simulink model "ATABEY_Model_sim"  (R2025b)
settings: Solver=VariableStepAuto  StartTime=0.0  StopTime=simTime  RelTol=1e-3
undefined symbols (not defined in the file or in its folder): x0
libraries: aerolibfltsims x2, instrumentseriallib x2, slpidlib x1
settings Model: Creator=erayacikgz  LastModifiedBy=Qeyosa

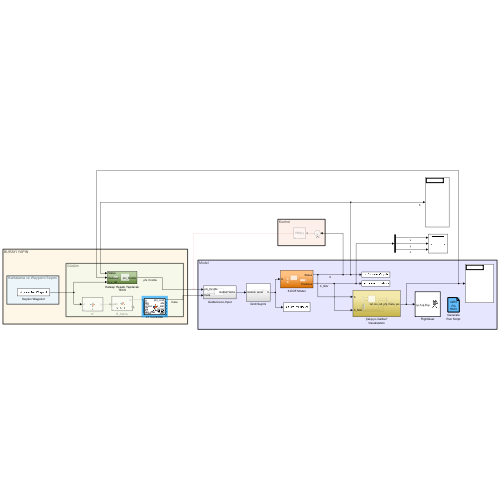
[thumbnail: Simulink's stored preview of the top-level diagram]
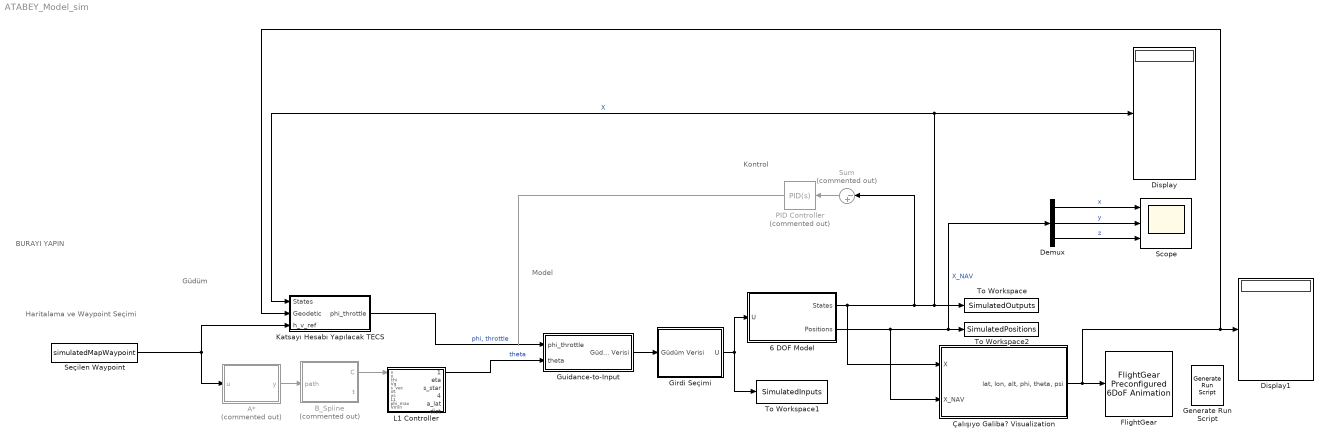
== system ATABEY_Model_sim ==
  note: BURAYI YAPIN
  note: Kontrol
  note: Haritalama ve Waypoint Seçimi
  note: Güdüm
  note: Model
  6 DOF Model : Subsystem
  A* : MATLAB Function  Commented=on  TreatAsAtomicUnit=on
  B_Spline : MATLAB Function  Commented=on  TreatAsAtomicUnit=on
  Demux : Demux  Outputs=3
  Display : Display
  Display1 : Display
  "FlightGear " : aerolibfltsims/FlightGear Preconfigured 6DoF Animation  xFlightGearVersion=v2019.1  DestinationIpAddress=127.0.0.1  DestinationPort=5502  SampleTime=1/30  packetVersion=24
  Generate Run Script : aerolibfltsims/Generate Run Script  Architecture=Linux  dataFlow=Send  GeometryModelName=c172p  AirportId=KSFO  RunwayId=10L  InitialAltitude=7224  InitialHeading=113  OffsetDistance=4.72  OffsetAzimuth=0  InstallScenery=off  DisableShaders=on  OriginAddress=127.0.0.1  DestinationPort=5502  OriginPort=5505  LocalAddress=127.0.0.1  OutputFileName=runfg.sh  FlightGearBaseDirectory=/usr/share/games/flightgear/
  Girdi Seçimi : Subsystem
  Guidance-to-Input : Subsystem
  Katsayı Hesabı Yapılacak TECS : Subsystem
  L1 Controller : MATLAB Function  TreatAsAtomicUnit=on
  PID Controller : slpidlib/PID Controller  Commented=on  Controller=PID  Form=Parallel  TimeDomain=Continuous-time  UseExternalTs=off  SampleTime=-1  IntegratorMethod=Forward Euler  FilterMethod=Forward Euler  ControllerParametersSource=internal  P=1  I=1  UseKiTs=off  D=0  UseExternalDerivativeSource=off  N=100  UseFilter=on  TunerSelectOption=Transfer Function Based (PID Tuner App)  InitialConditionSource=internal  InitialConditionForIntegrator=0  InitialConditionForFilter=0  DifferentiatorICPrevScaledInput=0  ExternalReset=none  TrackingMode=off  Kt=1  LimitOutput=off  SatLimitsSource=internal  UpperSaturationLimit=inf  LowerSaturationLimit=-inf  LinearizeAsGain=on  AntiWindupMode=none  Kb=1  LimitIntegrator=off  UpperIntegratorSaturationLimit=inf  LowerIntegratorSaturationLimit=-inf  POutMin=[]  POutMax=[]  IOutMin=[]  IOutMax=[]  DOutMin=[]  DOutMax=[]  NOutMin=[]  NOutMax=[]  SumOutMin=[]  SumOutMax=[]  SaturationOutMin=[]  SaturationOutMax=[]  PParamMin=[]  PParamMax=[]  IParamMin=[]  IParamMax=[]  DParamMin=[]  DParamMax=[]  NParamMin=[]  NParamMax=[]  KbParamMin=[]  KbParamMax=[]  KtParamMin=[]  KtParamMax=[]  KbOutMin=[]  KbOutMax=[]  KtOutMin=[]  KtOutMax=[]  IntegratorOutMin=[]  IntegratorOutMax=[]  FilterOutMin=[]  FilterOutMax=[]  SumI1OutMin=[]  SumI1OutMax=[]  SumI2OutMin=[]  SumI2OutMax=[]  SumI3OutMin=[]  SumI3OutMax=[]  SumI4OutMin=[]  SumI4OutMax=[]  SumDOutMin=[]  SumDOutMax=[]  DifferentiatorOutMin=[]  DifferentiatorOutMax=[]  FilterDiffOutCoefMin=[]  FilterDiffOutCoefMax=[]  ReciprocalOutMin=[]  ReciprocalOutMax=[]  SumDenOutMin=[]  SumDenOutMax=[]  SumNumOutMin=[]  SumNumOutMax=[]  DivideOutMin=[]  DivideOutMax=[]  UdiffTsProdOutMin=[]  UdiffTsProdOutMax=[]  NTsProdOutMin=[]  NTsProdOutMax=[]  UintegralTsProdOutMin=[]  UintegralTsProdOutMax=[]  UngainTsProdOutMin=[]  UngainTsProdOutMax=[]  ClampingZeroOutDataTypeStr=Inherit: Inherit via back propagation  ClampingZeroOutMin=[]  ClampingZeroOutMax=[]  FilterDenConstantOutDataTypeStr=Inherit: Inherit via back propagation  FilterDenConstantOutMin=[]  FilterDenConstantOutMax=[]  PCopyOutDataTypeStr=Inherit: Inherit via back propagation  PCopyOutMin=[]  PCopyOutMax=[]  NCopyOutDataTypeStr=Inherit: Inherit via back propagation  NCopyOutMin=[]  NCopyOutMax=[]  IntegratorContinuousStateAttributes=''  IntegratorStateMustResolveToSignalObject=off  IntegratorRTWStateStorageClass=Auto  FilterContinuousStateAttributes=''  FilterStateMustResolveToSignalObject=off  FilterRTWStateStorageClass=Auto  ParallelPVariant=InternalParameters  IdealPVariant=Disabled  IVariant=InternalParameters  DVariant=InternalParameters  IntegratorVariant=Continuous  SatVariant=Disabled  AWVariant=Passthrough  PCopyVariant=Disabled  TRVariant=Disabled  FdbkBlocksVariant=Forward  IdealPFdbkVariant=Disabled  SatFdbkVariant=Disabled  DerivativeFilterVariant=ContFilter  NVariant=InternalParameters  NCopyVariant=Disabled  FilterICVariant=InternalICsFilter  IntegratorICVariant=InternalICs  ExternalResetVariant=Disabled  TRSumVariant=Passthrough  SumFdbkVariant=Disabled  SumVariant=Sum_PID  TsampFilterVariant=InternalTs  TsampNgainVariant=Passthrough  TsampIntegralVariant=Disabled_SignalSpec  ExternalSaturationOutDataTypeStr=Inherit: Same as second input  DerivativeSourceVariant=ErrorSignal  PreIntVariant=InternalPreInt
  Scope : Scope  NumInputPorts=3
      settings: ActiveDisplayYMinimum=-216.60563593004551  ActiveDisplayYMaximum=141.28895348469339
  Seçilen Waypoint : FromWorkspace  VariableName=simulatedMapWaypoint
  Sum : Sum  Commented=on  Inputs=|-+
  To Workspace : ToWorkspace  VariableName=SimulatedOutputs  SaveFormat=Timeseries  SampleTime=-1
  To Workspace1 : ToWorkspace  VariableName=SimulatedInputs  SaveFormat=Timeseries  SampleTime=-1
  To Workspace2 : ToWorkspace  VariableName=SimulatedPositions  SaveFormat=Timeseries  SampleTime=-1
  Çalışıyo Galiba? Visualization : Subsystem
  wires:
  Çalışıyo Galiba? Visualization/1("lat, lon, alt, phi, theta, psi") -> Katsayı Hesabı Yapılacak TECS/2(Geodetic), Display1/1, "FlightGear "/1
  Guidance-to-Input/1(Güdüm Verisi) -> Girdi Seçimi/1(Güdüm Verisi)
  6 DOF Model/2(Positions) -> Demux/1, To Workspace2/1, Çalışıyo Galiba? Visualization/2(X_NAV)  "X_NAV"
  6 DOF Model/1(States) -> Sum/1, Display/1, Katsayı Hesabı Yapılacak TECS/1(States), To Workspace/1, Çalışıyo Galiba? Visualization/1(X)  "X"
  Demux/1 -> Scope/1  "x"
  Demux/2 -> Scope/2  "y"
  Demux/3 -> Scope/3  "z"
  Girdi Seçimi/1(U) -> To Workspace1/1, 6 DOF Model/1(U)
  Sum/1 -> PID Controller/1
  Katsayı Hesabı Yapılacak TECS/1(phi_throttle) -> Guidance-to-Input/1(phi_throttle)  "phi, throttle"
  Seçilen Waypoint/1 -> Katsayı Hesabı Yapılacak TECS/3(h_v_ref), A*/1(u)
  A*/1(y) -> B_Spline/1(path)
  B_Spline/1(C) -> L1 Controller/1(x)
  L1 Controller/1(phi_cmd) -> Guidance-to-Input/2(theta)  "theta"
  PID Controller/1 -> ?

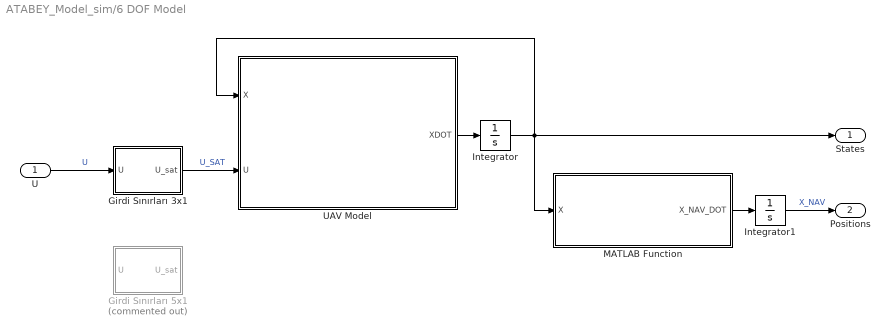
== system ATABEY_Model_sim/6 DOF Model ==
  U : Inport
  Girdi Sınırları 3x1 : Subsystem
  Girdi Sınırları 5x1 : Subsystem  Commented=on
  Integrator : Integrator  InitialCondition=x0(:,:)
  Integrator1 : Integrator  InitialCondition=[0;0;0;]
  MATLAB Function : MATLAB Function  TreatAsAtomicUnit=on
  UAV Model : MATLAB Function  TreatAsAtomicUnit=on
  States : Outport
  Positions : Outport  Port=2
  wires:
  Girdi Sınırları 3x1/1(U_sat) -> UAV Model/2(U)  "U_SAT"
  Integrator1/1 -> Positions/1  "X_NAV"
  MATLAB Function/1(X_NAV_DOT) -> Integrator1/1
  Integrator/1 -> MATLAB Function/1(X), States/1, UAV Model/1(X)
  UAV Model/1(XDOT) -> Integrator/1
  U/1 -> Girdi Sınırları 3x1/1(U)  "U"

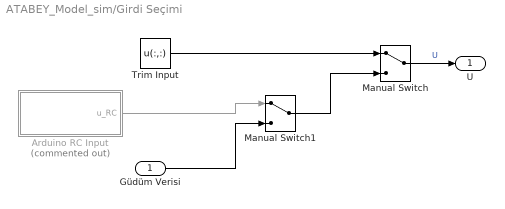
== system ATABEY_Model_sim/Girdi Seçimi ==
  Güdüm Verisi : Inport
  Arduino RC Input : Subsystem  Commented=on
  Manual Switch : ManualSwitch
  Manual Switch1 : ManualSwitch
  Trim Input : Constant  Value=u(:,:)
  U : Outport
  wires:
  Güdüm Verisi/1 -> Manual Switch1/2
  Manual Switch/1 -> U/1  "U"
  Arduino RC Input/1(u_RC) -> Manual Switch1/1
  Manual Switch1/1 -> Manual Switch/2
  Trim Input/1 -> Manual Switch/1

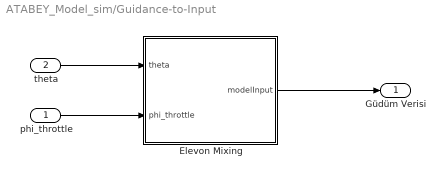
== system ATABEY_Model_sim/Guidance-to-Input ==
  phi_throttle : Inport
  theta : Inport  Port=2
  Elevon Mixing : MATLAB Function  TreatAsAtomicUnit=on
  Güdüm Verisi : Outport
  wires:
  Elevon Mixing/1(modelInput) -> Güdüm Verisi/1
  phi_throttle/1 -> Elevon Mixing/2(phi_throttle)
  theta/1 -> Elevon Mixing/1(theta)

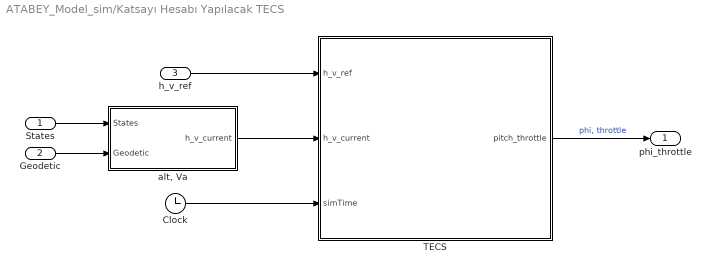
== system ATABEY_Model_sim/Katsayı Hesabı Yapılacak TECS ==
  States : Inport
  Geodetic : Inport  Port=2
  h_v_ref : Inport  Port=3
  Clock : Clock
  TECS : MATLAB Function  TreatAsAtomicUnit=on
  "alt, Va" : MATLAB Function  TreatAsAtomicUnit=on
  phi_throttle : Outport
  wires:
  h_v_ref/1 -> TECS/1(h_v_ref)
  Clock/1 -> TECS/3(simTime)
  "alt, Va"/1(h_v_current) -> TECS/2(h_v_current)
  TECS/1(pitch_throttle) -> phi_throttle/1  "phi, throttle"
  States/1 -> "alt, Va"/1(States)
  Geodetic/1 -> "alt, Va"/2(Geodetic)

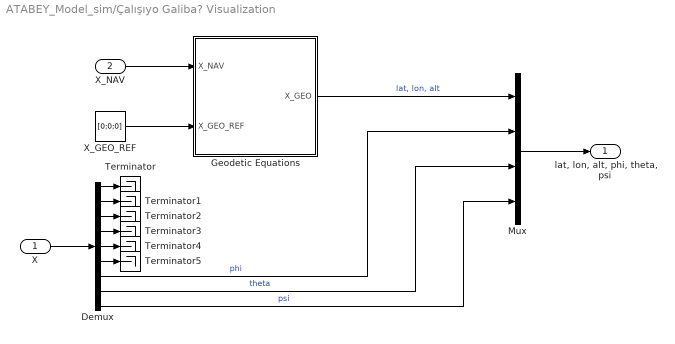
== system ATABEY_Model_sim/Çalışıyo Galiba? Visualization ==
  X : Inport
  X_NAV : Inport  Port=2
  Demux : Demux  Outputs=9
  Geodetic Equations : MATLAB Function  TreatAsAtomicUnit=on
  Mux : Mux
  Terminator{,1..5} (6 alike) : Terminator
  X_GEO_REF : Constant  Value=[0;0;0]
  "lat, lon, alt, phi, theta, psi" : Outport
  wires:
  Mux/1 -> "lat, lon, alt, phi, theta, psi"/1
  Geodetic Equations/1(X_GEO) -> Mux/1  "lat, lon, alt"
  Demux/9 -> Mux/4  "psi"
  Demux/7 -> Mux/2  "phi"
  X_NAV/1 -> Geodetic Equations/1(X_NAV)
  Demux/4 -> Terminator3/1
  X/1 -> Demux/1
  Demux/5 -> Terminator4/1
  X_GEO_REF/1 -> Geodetic Equations/2(X_GEO_REF)
  Demux/8 -> Mux/3  "theta"
  Demux/3 -> Terminator2/1
  Demux/2 -> Terminator1/1
  Demux/1 -> Terminator/1
  Demux/6 -> Terminator5/1

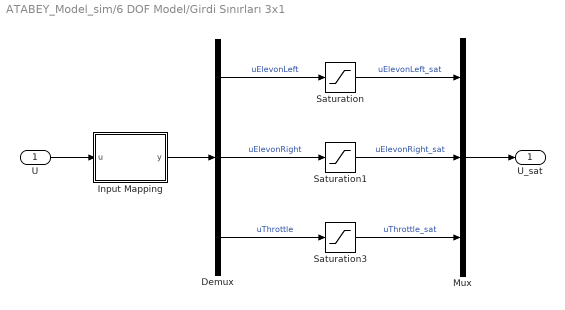
== system ATABEY_Model_sim/6 DOF Model/Girdi Sınırları 3x1 ==
  U : Inport
  Demux : Demux  Outputs=3
  Input Mapping : MATLAB Function  TreatAsAtomicUnit=on
  Mux : Mux  Inputs=3
  Saturation : Saturate  UpperLimit=20  LowerLimit=-20
  Saturation1 : Saturate  UpperLimit=20  LowerLimit=-20
  Saturation3 : Saturate  UpperLimit=1  LowerLimit=0
  U_sat : Outport
  wires:
  Saturation3/1 -> Mux/3  "uThrottle_sat"
  Demux/3 -> Saturation3/1  "uThrottle"
  Saturation1/1 -> Mux/2  "uElevonRight_sat"
  Demux/1 -> Saturation/1  "uElevonLeft"
  U/1 -> Input Mapping/1(u)
  Saturation/1 -> Mux/1  "uElevonLeft_sat"
  Demux/2 -> Saturation1/1  "uElevonRight"
  Mux/1 -> U_sat/1
  Input Mapping/1(y) -> Demux/1

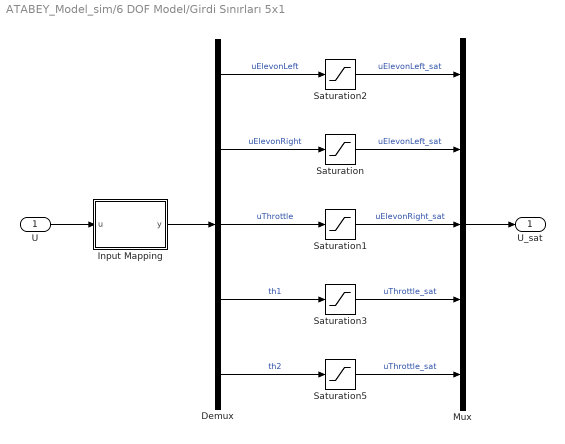
== system ATABEY_Model_sim/6 DOF Model/Girdi Sınırları 5x1 ==
  U : Inport
  Demux : Demux  Outputs=5
  Input Mapping : MATLAB Function  TreatAsAtomicUnit=on
  Mux : Mux  Inputs=5
  Saturation : Saturate  UpperLimit=20  LowerLimit=-20
  Saturation1 : Saturate  UpperLimit=20  LowerLimit=-20
  Saturation2 : Saturate  UpperLimit=20  LowerLimit=-20
  Saturation3 : Saturate  UpperLimit=1  LowerLimit=0
  Saturation5 : Saturate  UpperLimit=1  LowerLimit=0
  U_sat : Outport
  wires:
  U/1 -> Input Mapping/1(u)
  Mux/1 -> U_sat/1
  Input Mapping/1(y) -> Demux/1
  Demux/1 -> Saturation2/1  "uElevonLeft"
  Demux/2 -> Saturation/1  "uElevonRight"
  Demux/3 -> Saturation1/1  "uThrottle"
  Demux/4 -> Saturation3/1  "th1"
  Demux/5 -> Saturation5/1  "th2"
  Saturation2/1 -> Mux/1  "uElevonLeft_sat"
  Saturation/1 -> Mux/2  "uElevonLeft_sat"
  Saturation1/1 -> Mux/3  "uElevonRight_sat"
  Saturation3/1 -> Mux/4  "uThrottle_sat"
  Saturation5/1 -> Mux/5  "uThrottle_sat"

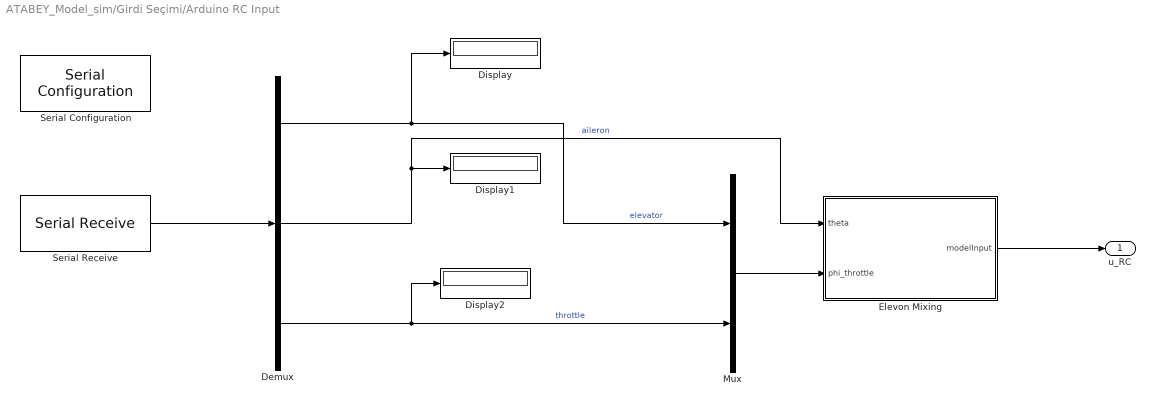
== system ATABEY_Model_sim/Girdi Seçimi/Arduino RC Input ==
  Demux : Demux  Outputs=3
  Display : Display
  Display1 : Display
  Display2 : Display
  Elevon Mixing : MATLAB Function  TreatAsAtomicUnit=on
  Mux : Mux  Inputs=2
  Serial Configuration : instrumentseriallib/Serial Configuration  Priority=-200000  PortSel=/dev/ttyUSB0  Port=/dev/ttyUSB0  ComPort=/dev/ttyUSB0  BaudRate=9600  DataBits=8  Parity=none  StopBits=1  ByteOrder=little-endian  FlowControl=none  Timeout=10  SimulateUsing=Interpreted execution  BlockInModel=on  aMode=1
      settings: LibrarySourceBlock=c2000lib/Host Communication/Serial Configuration
  Serial Receive : instrumentseriallib/Serial Receive  Priority=1  PortSel=/dev/ttyUSB0  Port=/dev/ttyUSB0  ComPort=/dev/ttyUSB0  DataType=int16  SaveDataType=uint8  ToggleHeader=on  Header=[255]  ToggleDataSize=on  DataSize=[1 3]  ToggleTerminator=off  Terminator=<none>  CustomTerminator=[]  InputFormat=Column major  EnableBlockingMode=on  ActionDataUnavailable=Output last received value  ActionWhenDataUnavailable=Output last received value  CustomValue=0  SampleTime=0.01  SimulateUsing=Interpreted execution  BlockInModel=on  aMode=1  LibraryInUse=c2000lib
      settings: LibrarySourceBlock=c2000lib/Host Communication/Serial Receive
  u_RC : Outport
  wires:
  Serial Receive/1 -> Demux/1
  Demux/3 -> Display2/1, Mux/2  "throttle"
  Demux/1 -> Mux/1, Display/1  "elevator"
  Demux/2 -> Elevon Mixing/1(theta), Display1/1  "aileron"
  Elevon Mixing/1(modelInput) -> u_RC/1
  Mux/1 -> Elevon Mixing/2(phi_throttle)

== matlab function ATABEY_Model_sim/6 DOF Model/Girdi Sınırları 3x1/Input Mapping ==
  data: u input; y output
function y = fcn(u)

% Map first two values from [-100, 100] to [-20, 20]
y1 = double(u(1)) * (20 / 100);
y2 = double(u(2)) * (20 / 100);

% Map last value from [0, 100] to [0, 1]
y3 = double(u(end)) * (1 / 100);

y = [y1; y2; y3];

== matlab function ATABEY_Model_sim/6 DOF Model/Girdi Sınırları 5x1/Input Mapping ==
  data: u input; y output
function y = fcn(u)

% Map first two values from [-100, 100] to [-20, 20]
y1 = double(u(1)) * (20 / 100);
y2 = double(u(2)) * (20 / 100);

% Map last value from [0, 100] to [0, 1]
y3 = double(u(end)) * (1 / 100);

y = [y1; y2; y3];

== matlab function ATABEY_Model_sim/Katsayı Hesabı Yapılacak TECS/alt, Va ==
  data: States input; h_v_current output; Geodetic input
function h_v_current = fcn(States, Geodetic)

% Modelden ve Navigasyon Hesaplarından İrtifa ve Hız Çek

alt = Geodetic(3);

u = States(1); v = States(2); w = States(3);
Va = sqrt(u^2 + v^2 + w^2);

h_v_current = [alt,Va];

== matlab function ATABEY_Model_sim/6 DOF Model/MATLAB Function ==
  data: X input; X_NAV_DOT output
function X_NAV_DOT  = NavigationEquations(X)

P_N_dot = X(1)*cos(X(8))*cos(X(9))...
    + X(2)*(-cos(X(7))*sin(X(9)) + sin(X(7))*sin(X(8))*cos(X(9)))...
    + X(3)*(sin(X(7))*sin(X(9)) + cos(X(7))*sin(X(8))*cos(X(9)));

P_E_dot = X(1)*cos(X(8))*sin(X(9))...
    + X(2)*(cos(X(7))*cos(X(9)) + sin(X(7))*sin(X(8))*sin(X(9)))...
    + X(3)*(-sin(X(7))*cos(X(9)) + cos(X(7))*sin(X(8))*sin(X(9)));

h_dot = X(1)*sin(X(8)) - X(2)*sin(X(7))*cos(X(8)) - X(3)*cos(X(7))*cos(X(8));

X_NAV_DOT = [P_N_dot;
             P_E_dot;
             h_dot];

end

== matlab function ATABEY_Model_sim/6 DOF Model/UAV Model ==
  data: X input double size=[9 1]; XDOT output double size=[9 1]; U input double
% MATLAB/ATABEY_dynamics
% Fonksiyon, dinamik dosyasını çağırır, modüler değişiklik yapmak için

function XDOT = ATABEY_model(X, U)

    XDOT = ATABEY_dynamics(X, U);

end

== matlab function ATABEY_Model_sim/Çalışıyo Galiba? Visualization/Geodetic Equations ==
  data: X_NAV input; X_GEO output; X_GEO_REF input
function X_GEO = FlatEarthtoGeodetic(X_NAV, X_GEO_REF)

PN = X_NAV(1);               % Kuzey (m)
PE = X_NAV(2);               % Doğu  (m)
PH = X_NAV(3);               % Positive Down

lat0 = X_GEO_REF(1);
lon0 = X_GEO_REF(2);
alt0 = X_GEO_REF(3);

% WGS-84
a = 6378137.0;               % Semi-major axis (m)
f = 1/298.257223563;         % Flattening
e2 = 2*f - f^2;              % Eccentricity squared

lat0_rad = deg2rad(lat0);

% Eğri Yarıçapı, Prime Vertical
N = a / sqrt(1 - e2 * sin(lat0_rad)^2);

% Eğri Yarıçapı, Meridyen
M = a * (1 - e2) / (1 - e2 * sin(lat0_rad)^2)^1.5;

% PN/PE -> delta lat/lon (rad)
d_lat = PN / M;
d_lon = PE / (N * cos(lat0_rad));

% Çıktı
lat = lat0 + rad2deg(d_lat); % deg
lon = lon0 + rad2deg(d_lon); % deg
alt = -1*(alt0 - PH);             % m

X_GEO = [lat,lon,alt];

end

== matlab function ATABEY_Model_sim/A* ==
  data: u input; y output
function y = fcn(u)

y = u;

== matlab function ATABEY_Model_sim/B_Spline ==
  data: path input; C output; t output
function [C, t] = B_Spline(path)
% Inputs:
%   path - A* result [n x 2] or [n x 3] of [row, col] grid indices
k = 4;      % Spline order (degree = k-1). Default: 4 (cubic)
n = 500;    % Number of output curve points. Default: 500
%
% Outputs:
%   C    - Evaluated curve points [n x d]  <-- feed this to L1
  % t    - Parameter values [1 x n]

% Defaults
if nargin < 2, k = 4;   end
if nargin < 3, n = 500; end

%% A* -> Control Points
P = double(path);

if iscolumn(P) && size(P, 2) == 1
    error('path_to_bspline: path must be [n x 2] or [n x 3], not a linear index vector.');
end

% Remove consecutive duplicates (prevents zero-length knot spans)
mask = [true; any(diff(P, 1, 1) ~= 0, 2)];
P    = P(mask, :);

% [row, col] -> [x, y]  (comment out if A* already returns [x, y])
P = fliplr(P);

%% Evaluate B-Spline
[m, d]    = size(P);
num_knots = m + k;

% Clamped uniform knot vector
knots = [zeros(1, k), linspace(0, 1, num_knots - 2*k + 2), ones(1, k)];

t = linspace(knots(k), knots(m + 1), n);
C = zeros(n, d);

for i = 1:n
    % de Boor evaluation at t(i)
    ti = t(i);

    % Knot span index
    if ti == knots(end)
        r = m;
    else
        r = min(find(knots <= ti, 1, 'last') - 1, m);
    end

    % Local control points for this span
    idx = max(1, min((r - k + 1):r, m));
    dp  = P(idx, :);

    % de Boor recursion
    for s = 1:(k - 1)
        for j = k:-1:(s + 1)
            i_knot = r - k + j;
            denom  = knots(i_knot + k - s) - knots(i_knot);
            alpha  = 0;
            if denom ~= 0
                alpha = (ti - knots(i_knot)) / denom;
            end
            dp(j, :) = (1 - alpha) * dp(j - 1, :) + alpha * dp(j, :);
        end
    end

    C(i, :) = dp(k, :);
end

end

== matlab function ATABEY_Model_sim/L1 Controller ==
  data: x input; phi_cmd output; y input; chi input; Vg input; s_vec input; xs input; ys input; L1 input; phi_max input; Vmin input; eta output; s_star output; s_target output; a_lat output; dist output
function [phi_cmd, eta, s_star, s_target, a_lat, dist] = L1_Controller(...
    x, y, chi, Vg, s_vec, xs, ys, L1, phi_max, Vmin)

% Girişler:
% x, y        : UAV pozisyonu
% chi         : Yönelim (rad)
% Vg          : Yere göre hız (m/s)
% s_vec       : Path parametre vektörü
% xs, ys      : Path koordinatları
% L1          : Lookahead distance
% phi_max     : Maksimum roll açısı
% Vmin        : Minimum hız 
%
% Çıkışlar:
% phi_cmd     : Roll komutu (rad)
% eta         : Heading hatası (rad) (debug)
% s_star      : Path üzerindeki en yakın nokta parametresi (debug)
% s_target    : Lookahead noktası parametresi (debug)
% a_lat       : Lateral ivme (m/s^2) (debug)
% dist        : Path'e olan mesafe (debug)


% 1 - SPEED CLAMP

if Vg < Vmin
    Vg = Vmin;
end

% 2 - CLOSEST POINT (Projection)

min_dist = 1e9;
s_star = s_vec(1);

for i = 1:length(s_vec)
    % Araç ve path noktası arasındaki mesafe hesaplanması
    dx = x - xs(i);
    dy = y - ys(i);

    % Kare mesafe (Karekök almamayı tercih ettim performans için)
    d = dx*dx + dy*dy;
    
    % Minimum mesafe güncellenmesi
    if d < min_dist
        min_dist = d;
        s_star = s_vec(i);
    end
end

% 3 - LOOKAHEAD POINT

s_target = s_star + L1;

% Path sınırı (boundary condition)
if s_target > s_vec(end)
    s_target = s_vec(end);
end

% Lineer İnterpolasyon (s_target tam grid olmayabilir. Ara değeri alalım)
x_L1 = interp1(s_vec, xs, s_target);
y_L1 = interp1(s_vec, ys, s_target);

% 4 - VECTOR COMPUTATION

% L1 - UAV vektörü
L1x = x_L1 - x;
L1y = y_L1 - y;

% UAV'nin yere göre hız vektörü
Vgx = Vg * cos(chi);
Vgy = Vg * sin(chi);

% 5 - ETA ANGLE

% UAV güncel yön ve aslında olması gereken yön arasındaki açı farkı
cross = Vgx * L1y - Vgy * L1x;
dot   = Vgx * L1x + Vgy * L1y;
eta = atan2(cross, dot);

% 6 - L1 GUIDANCE

a_lat = 2 * Vg^2 / L1 * sin(eta);


% 7 - ROLL COMMAND

% a_lat değeri roll açısına döndürülür.
g = 9.81;
phi_cmd = atan(a_lat / g);


% 8 - SATURATION

% Verilen komutların uçağın fiziksel sınırları arasında kalmasını
% garantilemek için gerekli kod bloğu
if phi_cmd > phi_max
    phi_cmd = phi_max;
elseif phi_cmd < -phi_max
    phi_cmd = -phi_max;
end

end

== matlab function ATABEY_Model_sim/Katsayı Hesabı Yapılacak TECS/TECS ==
  data: h_v_ref input; h_v_current input; pitch_throttle output; simTime input
function pitch_throttle  = TECS( ...
    h_v_ref, ...                    % Referans irtifa (m), hız (m/s)
    h_v_current, ...                % Mevcut irtifa (m), hız (m/s)
    simTime)

% Integralleri başlat
persistent int_E int_B
if isempty(int_E)
    int_E = 0;
end
if isempty(int_B)
    int_B = 0;
end

% Fonksiyon frekansını simülasyon frekansına eşitleme
persistent t_prev               
if isempty(t_prev)
    t_prev = simTime;
end

dt = simTime - t_prev;
t_prev = simTime;

%% GİRDİLER
mass = 2.5; g = 9.81;       % Araç kütlesi, yerçekimi ivmesi
Kp_E = 1; Ki_E = 1;         % Total Energy katsayılar
Kp_B = 1; Ki_B = 1;         % Energy Balance katsayılar

altitude_ref = h_v_ref(1); airspeed_ref = h_v_ref(2);
altitude_current = h_v_current(1); airspeed_current = h_v_current(2);

%% ENERJİ HESAPLARI

% Total Energy (E = mgh + 1/2 mV^2)
E     = mass * g * altitude_current     + 0.5 * mass * airspeed_current^2;
E_ref = mass * g * altitude_ref + 0.5 * mass * airspeed_ref^2;
E_err = E_ref - E; % Energy error

% Energy Balance (Potansiyel ve kinetik enerji arasındaki fark)
B     = mass * g * altitude_current     - 0.5 * mass * airspeed_current^2;
B_ref = mass * g * altitude_ref - 0.5 * mass * airspeed_ref^2;
B_err = B_ref - B; % Balance error

%% INTEGRAL HESABI
int_E = int_E + E_err * dt;
int_B = int_B + B_err * dt;

%% PI KONTROL

% Throttle controls TOTAL ENERGY
throttle_cmd = Kp_E * E_err + Ki_E * int_E;

% Pitch controls ENERGY BALANCE
pitch_cmd = Kp_B * B_err + Ki_B * int_B;

%% SATURASYON
% Throttle (0-1)
throttle_cmd = min(max(throttle_cmd, 0), 1);

% Pitch (rad)
pitch_max = deg2rad(20);
pitch_cmd = min(max(pitch_cmd, -pitch_max), pitch_max);

pitch_throttle = [pitch_cmd throttle_cmd];

end

== matlab function ATABEY_Model_sim/Guidance-to-Input/Elevon Mixing ==
  data: theta input; modelInput output; phi_throttle input
function modelInput  = elevonMix(theta, phi_throttle)
    phi = phi_throttle(1);
    
    % Elevon mixing
    elevon_left  = theta + phi;
    elevon_right = theta - phi;

    % % Clamp to actuator limits 
    % -> Gerek yok gibi?
    % elevon_left  = max(-1.0, min(1.0, elevon_left));
    % elevon_right = max(-1.0, min(1.0, elevon_right));

    % Throttle passthrough
    throttle_out = phi_throttle(2);

    modelInput = [elevon_left;elevon_right;throttle_out];

end

== matlab function ATABEY_Model_sim/Girdi Seçimi/Arduino RC Input/Elevon Mixing ==
  data: theta input; modelInput output; phi_throttle input
function modelInput  = elevonMix(theta, phi_throttle)
    phi = phi_throttle(1);
    
    % Elevon mixing
    elevon_left  = theta + phi;
    elevon_right = theta - phi;

    % % Clamp to actuator limits 
    % -> Gerek yok gibi?
    % elevon_left  = max(-1.0, min(1.0, elevon_left));
    % elevon_right = max(-1.0, min(1.0, elevon_right));

    % Throttle passthrough
    throttle_out = phi_throttle(2);

    modelInput = [elevon_left;elevon_right;throttle_out];

end
